simulink model "Wheel"  (R2020a)
settings: Solver=VariableStepAuto  StartTime=0.0  StopTime=10.0  RelTol=1e-3
values from neighbouring files (symbols this model uses):
  Effective_radius = 0.2    [Properties.sldd]
settings Model: DataDictionary=Properties.sldd  Creator=Matthew  LastModifiedBy=Matthew
settings ModelReferenceCC: ModelReferenceMinAlgLoopOccurrences=on

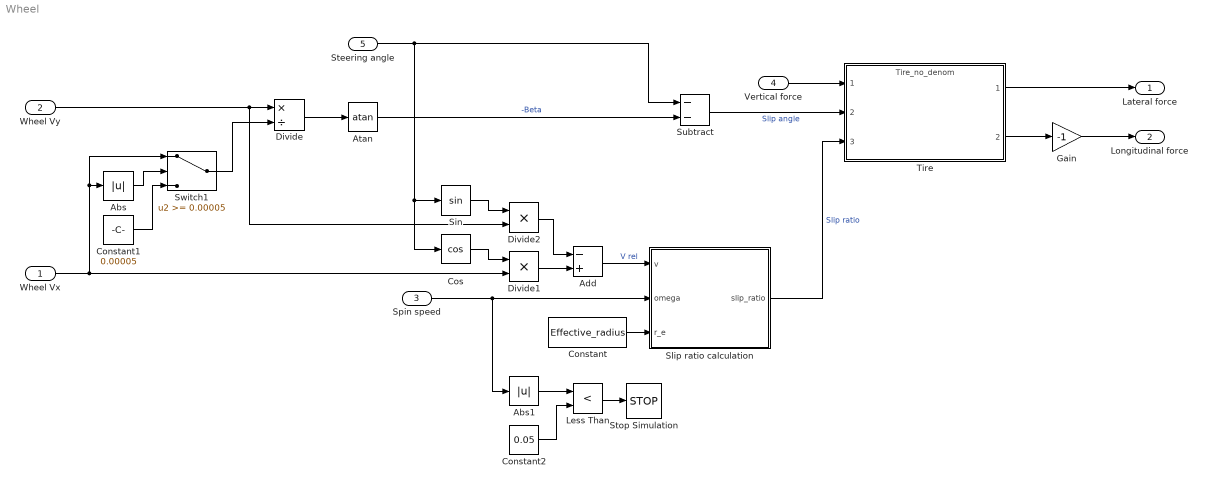
== system Wheel ==
  Wheel Vx : Inport
  Wheel Vy : Inport  Port=2
  Spin speed : Inport  Port=3
  Vertical force : Inport  Port=4
  Steering angle : Inport  Port=5
  Abs : Abs
  Abs1 : Abs
  Add : Sum  Inputs=-+
  Atan : Trigonometry  Operator=atan
  Constant : Constant  Value=Effective_radius
  Constant1 : Constant  Value=0.00005
  Constant2 : Constant  Value=0.05
  Cos : Trigonometry  Operator=cos
  Divide : Product  Inputs=*/
  Divide1 : Product  Inputs=**
  Divide2 : Product  Inputs=**
  Gain : Gain  Gain=-1
  Less Than : RelationalOperator  Operator=<  OutDataTypeStr=boolean  RndMeth=Simplest
  Sin : Trigonometry
  Slip ratio calculation : MATLAB Function
  Stop Simulation : Stop
  Subtract : Sum  Inputs=--
  Switch1 : Switch  Threshold=0.00005
  Tire : ModelReference  ModelNameDialog=Tire_no_denom.slx  SimulationMode=Normal  ModelReferenceVersion=1.22
  Lateral force : Outport
  Longitudinal force : Outport  Port=2
  wires:
  Slip ratio calculation/1(slip_ratio) -> Tire/3  "Slip ratio"
  Vertical force/1 -> Tire/1
  Subtract/1 -> Tire/2  "Slip angle"
  Spin speed/1 -> Abs1/1, Slip ratio calculation/2(omega)
  Tire/2 -> Gain/1
  Tire/1 -> Lateral force/1
  Wheel Vy/1 -> Divide2/2, Divide/1
  Divide/1 -> Atan/1
  Steering angle/1 -> Subtract/1, Cos/1, Sin/1
  Atan/1 -> Subtract/2  "-Beta"
  Constant/1 -> Slip ratio calculation/3(r_e)
  Add/1 -> Slip ratio calculation/1(v)  "V rel"
  Divide2/1 -> Add/1
  Divide1/1 -> Add/2
  Sin/1 -> Divide2/1
  Cos/1 -> Divide1/1
  Gain/1 -> Longitudinal force/1
  Switch1/1 -> Divide/2
  Abs/1 -> Switch1/2
  Wheel Vx/1 -> Divide1/2, Switch1/1, Abs/1
  Constant1/1 -> Switch1/3
  Abs1/1 -> Less Than/1
  Constant2/1 -> Less Than/2
  Less Than/1 -> Stop Simulation/1

== matlab function Wheel/Slip ratio calculation ==
  data: v input; slip_ratio output; omega input; r_e input
function slip_ratio = slip_ratio(v, omega, r_e)

if v > -0.005 && v < 0.005 && omega == 0 % Both are 0
    slip_ratio = 0;
elseif v > -0.005 && v < 0.005 % Only v is 0
    if omega > 0
        slip_ratio = 10;
    else
        slip_ratio = -10;
    end
else
    slip_ratio = (omega*r_e-v)/v; % v is non-zero
end
end
